simulink model "ConvolucionDiscretaSimulink"  (R2023b)
settings: Solver=FixedStepAuto  StartTime=0.0  StopTime=0.1  FixedStep=Ts  RelTol=1e-3
undefined symbols (not defined in the file): filtro, Ts

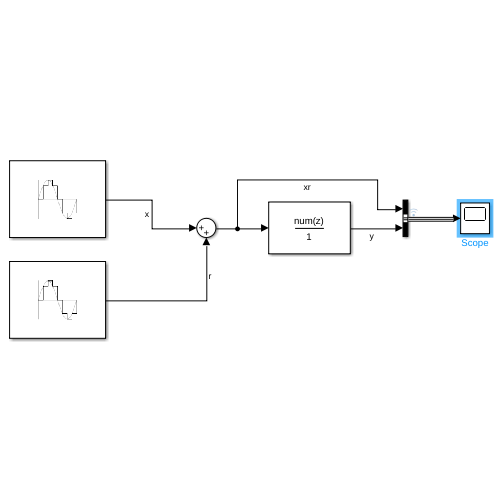
[thumbnail: Simulink's stored preview of the top-level diagram]
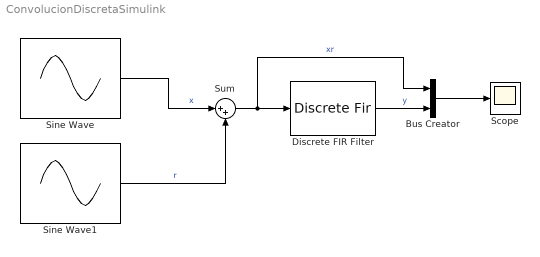
== system ConvolucionDiscretaSimulink ==
  Bus Creator : BusCreator  Inputs=2
  Discrete FIR Filter : DiscreteFir  Coefficients=filtro.Coefficients
  Scope : Scope
  Sine Wave : Sin  Amplitude=10  Frequency=2*pi*60  SampleTime=Ts
  Sine Wave1 : Sin  Amplitude=2.5  Frequency=2*pi*400  SampleTime=Ts
  Sum : Sum  Inputs=|++
  wires:
  Sine Wave/1 -> Sum/1  "x"
  Sine Wave1/1 -> Sum/2  "r"
  Sum/1 -> Bus Creator/1, Discrete FIR Filter/1  "xr"
  Discrete FIR Filter/1 -> Bus Creator/2  "y"
  Bus Creator/1 -> Scope/1
